simulink model "PID_0612"  (R2016b)
settings: Solver=VariableStepAuto  StartTime=0.0  StopTime=10  RelTol=1e-3
settings Model: Creator=xuzong  LastModifiedBy=xuzong

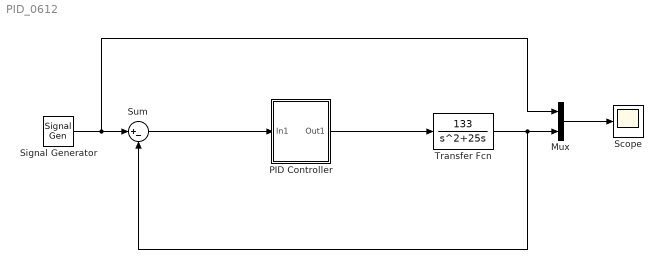
== system PID_0612 ==
  Mux : Mux  Inputs=2
  PID Controller : Subsystem
      mask Display: disp('PID\nController')
  Scope : Scope
  Signal Generator : SignalGenerator  WaveForm=square  Frequency=0.2
  Sum : Sum  Inputs=|+-
  Transfer Fcn : TransferFcn  Numerator=[133]  Denominator=[1 25 0]
  wires:
  Mux/1 -> Scope/1
  Transfer Fcn/1 -> Sum/2, Mux/2
  Signal Generator/1 -> Mux/1, Sum/1
  Sum/1 -> PID Controller/1(In1)
  PID Controller/1(Out1) -> Transfer Fcn/1

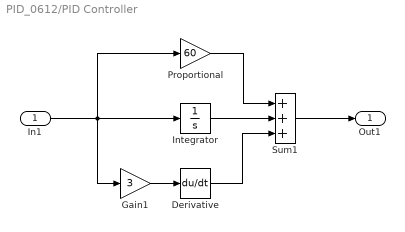
== system PID_0612/PID Controller ==
  In1 : Inport
  Derivative : Derivative
  Gain1 : Gain  Gain=3
  Integrator : Integrator
  Proportional : Gain  Gain=60
  Sum1 : Sum  Inputs=+++
  Out1 : Outport
  wires:
  In1/1 -> Proportional/1, Gain1/1, Integrator/1
  Proportional/1 -> Sum1/1
  Gain1/1 -> Derivative/1
  Sum1/1 -> Out1/1
  Integrator/1 -> Sum1/2
  Derivative/1 -> Sum1/3
